simulink model "AIE_HLS_clipping"  (R2021a)
settings: Solver=VariableStepAuto  StartTime=0.0  StopTime=inf  RelTol=1e-3
InitFcn:
  | load filter_coeffs.mat
  | LPF = round(LPF * 2^15)
undefined symbols (not defined in the file): S, vsva2197, xcvc1902
libraries: aieBasic x3, aieDSP x2, aieUtilities x2, dsparch4 x1, vmcUtilities x1, hlsBasic x1
settings Model: Creator=abehbood  LastModifiedBy=abehbood

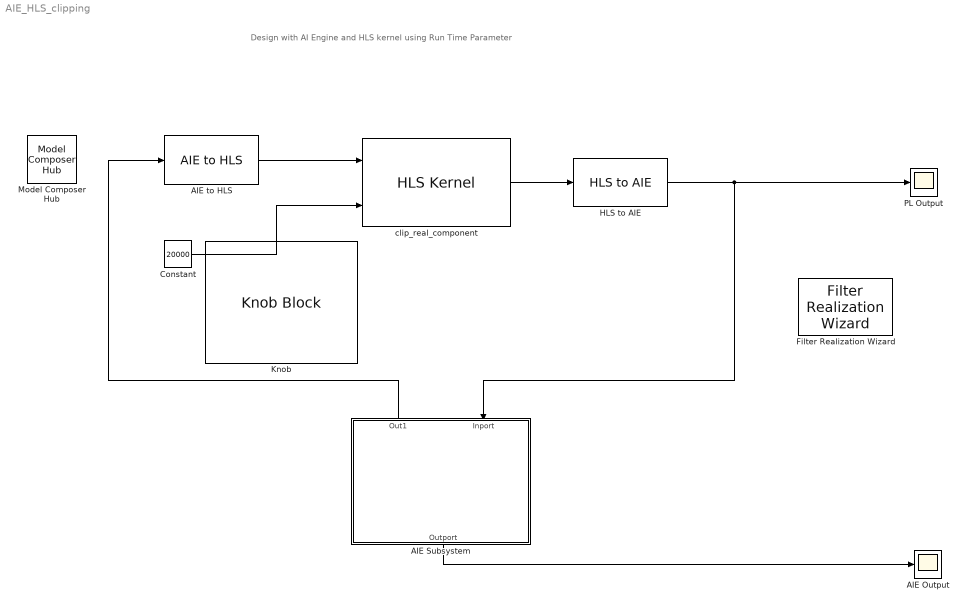
== system AIE_HLS_clipping ==
  note: Design with AI Engine and HLS kernel
      | using Run Time Parameter
  AIE Output : Scope
  AIE Subsystem : Subsystem
      settings: PortSchema="{\"entries\":[{\"content\":{\"sides\":[{\"content\":{\"connectorIds\":[\"Out2\"]},\"type\":\"ConnectorPlacement.EquallySpacedRectSide\",\"uuid\":\"600439e9-73c3-433c-a4a4-c36b72988664\"},{\"content\":{\"connectorIds\":[\"Out1\",\"In1\"],\"side\":\"RIGHT\"},\"type\":\"ConnectorPlacement.EquallySpacedRectSide\",\"uuid\":\"c5ca9a85-0742-44d8-b50a-7698103ab251\"},{\"content\":{\"connectorIds\":[],\"side\":\"TOP\"},\"type\":\"ConnectorPlacement.EquallySpacedRectSide\",\"uuid\":\"fb61f941-2da5-44dc-abf4-df4618bee3ad\"},{\"content\":{\"connectorIds\":[],\"side\":\"BOTTOM\"},\"type\":\"ConnectorPlacement.EquallySpacedRectSide\",\"uuid\":\"5a66f69a-5526-4d5e-a2d5-c31759d47fa6\"}]},\"type\":\"ConnectorPlacement.EquallySpacedConnector\",\"uuid\":\"81997a57-f7dc-4123-9425-e160d8e12fe0\"}],\"packageUris\":[\"http://schema.mathworks.com/mf0/Connector/R2020b\"],\"version\":\"1.0\"}"
  AIE to HLS : aieUtilities/AIE to HLS  OutputType=cint16  OutputSize=32
  Constant : Constant  Value=20000  OutDataTypeStr=int32  SampleTime=-1
  Filter Realization Wizard : dsparch4/Filter Realization Wizard
      settings: SourceProductBaseCode=DS
  HLS to AIE : aieUtilities/HLS to AIE  OutputType=cint16  OutputSize=32
  Knob : KnobBlock  LabelPosition=Hide  ScaleMin=20000  ScaleMax=32767
  Model Composer Hub : vmcUtilities/Model Composer Hub  Tag=genX  CodeGeneration=off  SubsystemName=AIE Subsystem  TargetDirectory=./code  ExportType=AI Engines  IpVendor=xilinx.com  IpLibrary=hls  IpVersion=1.0  IpHWLanguage=Verilog  AieCompilerOptions={}  CreateTestbench=on  TestbenchStackSize=10  RunAieSim=on  AieSimTimeout=5000  RunAieSimProfiling=off  LaunchVitisAnalyzer=off  PlotOutput=off  RunX86Sim=off  X86SimTimeout=10  GenHwImage=off  PlatformType=Not Specified  HwSystemType=Baremetal  HwValidationTarget=hw  ProjDevice=xcvc1902-vsva2197-2MP-e-S  ProjDevicePart=xcvc1902-vsva2197-2MP-e-S  SamplePeriod=-1  ClockFrequency=200  DataPathParallelism=1  xilinxfamily=Kintex7  part=xc7k325t  speed=-3  package=fbg676  directory=./netlist  testbench=off  incr_netlist=off  synthesis_tool=Vivado  clock_wrapper=Clock Enables  dbl_ovrd=According to Block Masks  dcm_input_clock_period=10  sysclk_period=10  simulink_period=1  eval_field=0
  PL Output : Scope
  clip_real_component : hlsBasic/HLS Kernel  PortNames={'return'; 'vin'; 'threshold'; 'vout'}  PortSerializedTypes={'{Bv}'; '{R{Thls::stream{2{t{Tstd::complex{1{t{Bi16}}}}}{t{}0}}}}'; '{Bi32}'; '{R{Thls::stream{2{t{Tstd::complex{1{t{Bi16}}}}}{t{}0}}}}'}  FunctionTemplateSpecKind=none  FunctionTemplateParamNames={}  FunctionTemplateParamKinds={}  FunctionTemplateParamTypes={}  FunctionTemplateParamValues={}  PortSynchronicities={'auto'; 'async'; 'auto'}  PortSignalSizes={0.000000000000000000e+00; 0.000000000000000000e+00; 3.200000000000000000e+01}  FunctionTemplateParams={}  FunctionTemplateParamsEnables={}  FunctionTemplateParamsVisible=off  FunctionDeclTypeOptions=C[1 1]@t7@<empty>  PortAttributesTable={ 'Input', 'vin', 'hls::stream< std::complex< int16 >, 0 > &', '', ''; 'Input', 'threshold', 'int32', 'async', ''; 'Output', 'vout', 'hls::stream< std::complex< int16 >, 0 > &', '', '32' }  PortAttributesEnablement={'off', 'off', 'off', 'off', 'off';'off', 'off', 'off', 'on', 'off';'off', 'off', 'off', 'off', 'on'}  SampleTime=-1  PortDirectionTable={ 'vin', 'hls::stream< std::complex< int16 >, 0 > &', 'Input'; 'threshold', 'int32', 'Input'; 'vout', 'hls::stream< std::complex< int16 >, 0 > &', 'Output' }  PortDirectionTabVisible=on  ArgDirections={1.000000000000000000e+00; 1.000000000000000000e+00; 2.000000000000000000e+00}  FunctionIndex=1  FormalArgDecls={'hls::stream< std::complex< int16 >, 0 > & vin', 'int32 threshold', 'hls::stream< std::complex< int16 >, 0 > & vout'}  SimLibPath=''  FunctionTabVisible=on  FunctionDescription=void clipper(hls::stream< std::complex< int16 >, 0 > & vin, int32 threshold, hls::stream< std::complex< int16 >, 0 > & vout)  KernelHeaderFile=src/clipper.h  KernelFunction=clipper  KernelFunctionSelect=<empty>  KernelSourceFile=src/clipper.cpp  KernelSearchPaths={}  PreProcOptions={}  blockJsonConstraints=[]  deprecateConstraints=0
  wires:
  AIE to HLS/1 -> clip_real_component/1
  Constant/1 -> clip_real_component/2
  clip_real_component/1 -> HLS to AIE/1
  AIE Subsystem/1(Out1) -> AIE to HLS/1
  AIE Subsystem/2(Outport) -> AIE Output/1
  HLS to AIE/1 -> AIE Subsystem/1(Inport), PL Output/1

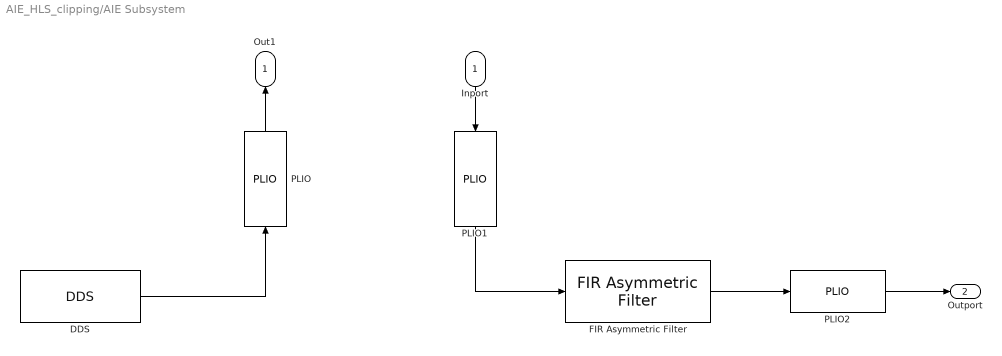
== system AIE_HLS_clipping/AIE Subsystem ==
  Inport : Inport
  DDS : aieDSP/DDS  data_type=cint16  output_window_size=32  phase_increment=2^25  vmc_sample_time=1  output_sampling_rate=200  spec=meta_data_hl_dds.json
  FIR Asymmetric Filter : aieDSP/FIR Asymmetric Filter  data_type=cint16  coef_type=int16  use_coeff_reload=off  coeff=LPF  fir_length=32  input_window_size=32  shift_val=16  rnd_mode=Round to positive infinity  input_sampling_rate=200  use_casc_length=on  casc_length=1  spec=meta_data_hl_fir_sr_asym.json
  PLIO : aieBasic/PLIO  PlioWidth=auto  PlioFreqSpec=off  PlioFreq=250  ColLocation=0  channel=0  blockJsonConstraints=[]  deprecateConstraints=0
  PLIO1 : aieBasic/PLIO  PlioWidth=auto  PlioFreqSpec=off  PlioFreq=250  ColLocation=0  channel=0  blockJsonConstraints=[]  deprecateConstraints=0
  PLIO2 : aieBasic/PLIO  PlioWidth=auto  PlioFreqSpec=off  PlioFreq=250  ColLocation=0  channel=0  blockJsonConstraints=[]  deprecateConstraints=0
  Out1 : Outport
  Outport : Outport  Port=2
  wires:
  DDS/1 -> PLIO/1
  PLIO/1 -> Out1/1
  FIR Asymmetric Filter/1 -> PLIO2/1
  PLIO1/1 -> FIR Asymmetric Filter/1
  PLIO2/1 -> Outport/1
  Inport/1 -> PLIO1/1
